simulink model "ABS_simulation"  (R2024b)
settings: Solver=VariableStepAuto  StartTime=0.0  StopTime=10.0  RelTol=1e-3
values from neighbouring files (symbols this model uses):
  g = 9.81    [ABS_simulation.mat]
  I = 6    [ABS_simulation.mat]
  m = 75    [ABS_simulation.mat]
  R = 1.255    [ABS_simulation.mat]
  V0 = 44    [ABS_simulation.mat]
settings Model: Creator=USER  LastModifiedBy=USER

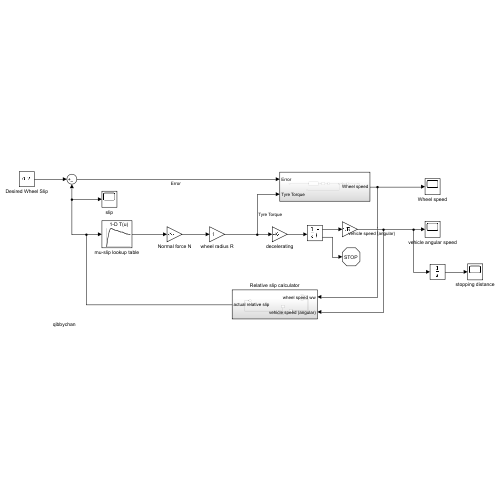
[thumbnail: Simulink's stored preview of the top-level diagram]
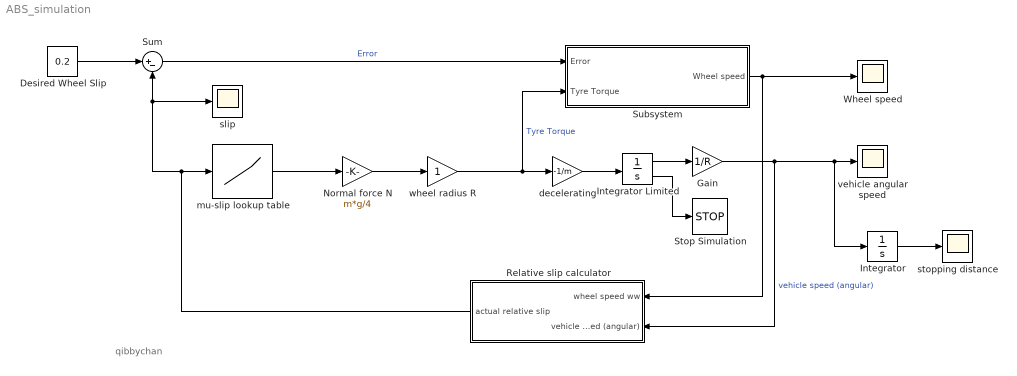
== system ABS_simulation ==
  note: qibbychan
  Desired Wheel Slip : Constant  Value=0.2
  Gain : Gain  Gain=1/R
  Integrator : Integrator
  Integrator Limited : Integrator  InitialCondition=V0  LimitOutput=on  UpperSaturationLimit=1000  LowerSaturationLimit=0  ShowSaturationPort=on
  Normal force N : Gain  Gain=m*g/4
  Relative slip calculator : Subsystem
  Stop Simulation : Stop
  Subsystem : Subsystem
  Sum : Sum  Inputs=|+-
  Wheel speed : Scope
  decelerating : Gain  Gain=-1/m
  mu-slip lookup table : Lookup_n-D  NumberOfTableDimensions=1  BreakpointsForDimension1=[0.00, 0.05, 0.10, 0.15, 0.20, 0.25, 0.30, 0.35, 0.40, 0.45, 0.50, 0.55, 0.60, 0.65, 0.70, 0.75, 0.80, 0.85, 0.90, 0.95, 1.00]  Table=[0.00, 0.42, 0.83, 0.96, 1.00, 0.97, 0.94, 0.91, 0.89, 0.87, 0.85, 0.83, 0.81, 0.79, 0.76, 0.74, 0.72, 0.70, 0.68, 0.66, 0.65]  InternalRulePriority=Speed  RndMeth=Simplest
  slip : Scope
  stopping distance : Scope
  vehicle angular speed : Scope
  wheel radius R : Gain
  wires:
  Desired Wheel Slip/1 -> Sum/1
  mu-slip lookup table/1 -> Normal force N/1
  Normal force N/1 -> wheel radius R/1
  Sum/1 -> Subsystem/1(Error)  "Error"
  wheel radius R/1 -> Subsystem/2(Tyre Torque), decelerating/1  "Tyre Torque"
  Subsystem/1(Wheel speed) -> Relative slip calculator/1(wheel speed ww), Wheel speed/1
  decelerating/1 -> Integrator Limited/1
  Integrator Limited/1 -> Gain/1
  Gain/1 -> vehicle angular speed/1, Integrator/1, Relative slip calculator/2(vehicle speed (angular))  "vehicle speed (angular)"
  Integrator Limited/2 -> Stop Simulation/1
  Integrator/1 -> stopping distance/1
  Relative slip calculator/1(actual relative slip) -> slip/1, Sum/2, mu-slip lookup table/1

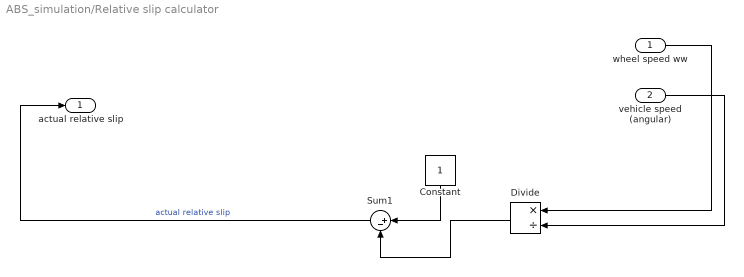
== system ABS_simulation/Relative slip calculator ==
  wheel speed ww : Inport
  vehicle speed (angular) : Inport  Port=2
  Constant : Constant
  Divide : Product  Inputs=*/
  Sum1 : Sum  Inputs=|+-
  actual relative slip : Outport
  wires:
  Divide/1 -> Sum1/2
  vehicle speed (angular)/1 -> Divide/2
  Constant/1 -> Sum1/1
  Sum1/1 -> actual relative slip/1  "actual relative slip"
  wheel speed ww/1 -> Divide/1

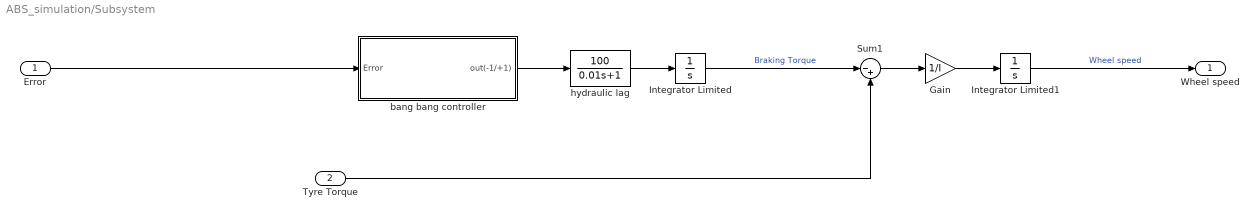
== system ABS_simulation/Subsystem ==
  Error : Inport
  Tyre Torque : Inport  Port=2
  Gain : Gain  Gain=1/I
  Integrator Limited : Integrator  InitialCondition=V0/R  LimitOutput=on  UpperSaturationLimit=1000  LowerSaturationLimit=0
  Integrator Limited1 : Integrator  InitialCondition=V0/R  LimitOutput=on  UpperSaturationLimit=1000  LowerSaturationLimit=0
  Sum1 : Sum  Inputs=|-+
  bang bang controller : Subsystem
  hydraulic lag : TransferFcn  Numerator=[100]  Denominator=[0.01 1]
  Wheel speed : Outport
  wires:
  Error/1 -> bang bang controller/1(Error)
  bang bang controller/1(out(-1/+1)) -> hydraulic lag/1
  Tyre Torque/1 -> Sum1/2
  hydraulic lag/1 -> Integrator Limited/1
  Integrator Limited/1 -> Sum1/1  "Braking Torque"
  Gain/1 -> Integrator Limited1/1
  Sum1/1 -> Gain/1
  Integrator Limited1/1 -> Wheel speed/1  "Wheel speed"

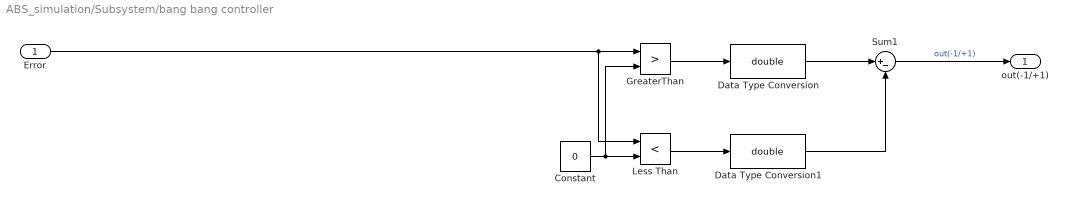
== system ABS_simulation/Subsystem/bang bang controller ==
  Error : Inport
  Constant : Constant  Value=0
  Data Type Conversion : DataTypeConversion  OutDataTypeStr=double  SaturateOnIntegerOverflow=off
  Data Type Conversion1 : DataTypeConversion  OutDataTypeStr=double  SaturateOnIntegerOverflow=off
  GreaterThan : RelationalOperator  Operator=>  OutDataTypeStr=boolean  RndMeth=Simplest  InputSameDT=off
  Less Than : RelationalOperator  Operator=<  OutDataTypeStr=boolean  RndMeth=Simplest  InputSameDT=off
  Sum1 : Sum  Inputs=|+-
  out(-1/+1) : Outport
  wires:
  GreaterThan/1 -> Data Type Conversion/1
  Error/1 -> Less Than/1, GreaterThan/1
  Constant/1 -> GreaterThan/2, Less Than/2
  Data Type Conversion1/1 -> Sum1/2
  Data Type Conversion/1 -> Sum1/1
  Less Than/1 -> Data Type Conversion1/1
  Sum1/1 -> out(-1/+1)/1  "out(-1/+1)"
